simulink subsystem "PvtSubSys_PLAN_DPC"  (R2020b)
settings: Solver=VariableStepAuto  StartTime=0.0  StopTime=10.0  RelTol=1e-3
undefined symbols (not defined in the file or in its folder): P_Global_DxvFrontBumper_m, P_Global_DxvRearBumper_m, P_PLAN_DPC_BrkPointDxFactorF1, P_PLAN_DPC_BrkPointDxFactorF2, P_PLAN_DPC_BrkPointDxFactorF3, P_PLAN_DPC_BrkPointDxFactorF4, P_PLAN_DPC_BrkPointDxFactorR1, P_PLAN_DPC_BrkPointDxFactorR2, P_PLAN_DPC_BrkPointDxFactorR3, P_PLAN_DPC_BrkPointDxFactorR4, P_PLAN_DPC_danqianleida_kaiguan, P_PLAN_DPC_danqianleida_maxDx, P_PLAN_DPC_danqianleida_minDx, P_PLAN_DPC_FrontObj_DX_00, P_PLAN_DPC_FrontObj_DX_03, P_PLAN_DPC_FrontObj_DX_08, P_PLAN_DPC_FrontObj_DX_1, P_PLAN_DPC_HearObj_DX_00, P_PLAN_DPC_HearObj_DX_03, P_PLAN_DPC_HearObj_DX_08, P_PLAN_DPC_HearObj_DX_11, P_PLAN_DPC_HWALineRearA2Factor, P_PLAN_DPC_HWALineRearA3Factor, P_PLAN_DPC_ObjAxLPalpha, P_PLAN_DPC_ObjDxLPalpha, P_PLAN_DPC_ObjDyLPalpha, P_PLAN_DPC_ObjVxLPalpha, P_PLAN_DPC_xiangduisudu_kmh
libraries: simulink x22
(part 1 of 3)
settings Model: Creator=GW00166368  LastModifiedBy=GW00180587

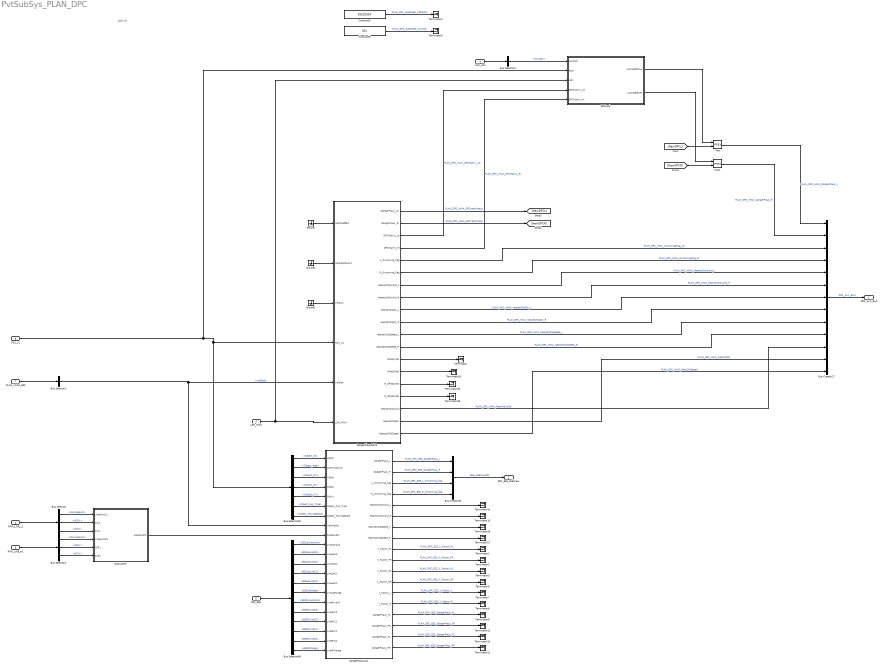
== system PvtSubSys_PLAN_DPC ==
  note: 变更记录
  VSM_HMI : Inport  Description=用了bus里面的HWASts，判断是否换道，用于锁止模块释放信号  OutDataTypeStr=Bus: VSM_HMI_BUS
  RFM_LINE_L1 : Inport  Description=本车道左车道线的属性用于计算车道宽度  Port=2  OutDataTypeStr=Bus: RFM_LINE_BUS
  RFM_LINE_R1 : Inport  Description=本车道右车道线的属性用于计算车道宽度  Port=3  OutDataTypeStr=Bus: RFM_LINE_BUS
  LSM_HWA : Inport  Description=|  Port=4  OutDataTypeStr=Bus: LSM_HWA_BUS
      | HWALeLineValid	boolean	1			HWA左目标线有效性
      | HWALeLineC3	single	1			HWA左目标线C3
      | HWALeLineC2	single	1			HWA左目标线C2
      | HWALeLineC1	single	1			HWA左目标线C1
      | HWALeLineC0	single	1			HWA左目标线C0
      | HWALeRange	single	1			HWA左目标线有效长度
      | HWALineValid	boolean	1			HWA目标线有效性
      | HWALineC3	single	1			HWA目标线C3
      | HWALineC2	single	1			HWA目标线C2
      | HWALineC1	single	1			HWA目标线C1
      | HWALineC0	single	1			HWA目标线C0
      | HWARange	single	1	m		HWA目标线有效长度
      | HWARiLineValid	boolean	1			HWA右目标线有效性
      | HWARiLineC3	single	1			HWA右目标线C3
      | HWARiLineC2	single	1			HWA右目标线C2
      | HWARiLineC1	single	1			HWA右目标线C1
      | HWARiLineC0	single	1			HWA右目标线C0
      | HWARiRange	single	1			HWA右目标线有效长度
  LSM_ESS : Inport  Description=|  Port=5  OutDataTypeStr=Bus: LSM_ESS_BUS
      | ESSLeLineValid	boolean	1			ESS左车道有效性
      | ESSLeLineC3	single	1			ESS左车道C3
      | ESSLeLineC2	single	1			ESS左车道C2
      | ESSLeLineC1	single	1			ESS左车道C1
      | ESSLeLineC0	single	1			ESS左车道C0
      | ESSLeRange	single	1			ESS左车道有效长度
      | ESSRiLineValid	boolean	1			ESS右车道有效性
      | ESSRiLineC3	single	1			ESS右车道C3
      | ESSRiLineC2	single	1			ESS右车道C2
      | ESSRiLineC1	single	1			ESS右车道C1
      | ESSRiLineC0	single	1			ESS右车道C0
      | ESSRiRange	single	1			ESS右车道有效长度
  TOS_LC : Inport  Description=|  Port=6  OutDataTypeStr=Bus: TOS_LC_BUS
      | Object_ID	single	(11,1)			障碍物ID。用于判断障碍物是否有效计算。
      | Object_DX	single	(11,1)			障碍物纵向距离。用于危险度计算。
      | Object_DY	single	(11,1)			障碍物横向距离。用于危险度计算。
      | Object_VX	single	(11,1)			障碍物纵向速度。用于危险度计算
  PLAN_VCAN_ESP : Inport  Description=自车车速  Port=7  OutDataTypeStr=Bus: VCAN_ESP_MSG_BUS
  Bus Creator17 : BusCreator  Inputs=13
  Bus Creator30 : BusCreator  Inputs=4
  Bus Selector : BusSelector  OutputSignals=bIsLineExist,dC0V,dC1V
  Bus Selector1 : BusSelector  OutputSignals=bIsLineExist,dC0V,dC1V
  Bus Selector2 : BusSelector  OutputSignals=VehSpd
  Bus Selector3 : BusSelector  OutputSignals=HWASts
  Bus Selector68 : BusSelector  OutputSignals=ESSLeLineValid,ESSLeLineC3,ESSLeLineC2,ESSLeLineC1,ESSLeLineC0,ESSLeRange,ESSRiLineValid,ESSRiLineC3,ESSRiLineC2,ESSRiLineC1,ESSRiLineC0,ESSRiRange
  Bus Selector82 : BusSelector  OutputSignals=Object_ID,Object_Age,Object_DX,Object_DY,Object_VX,Object_Fus_Type,Object_MovingState
  Constant5 : Constant  Value=39220304  OutDataTypeStr=uint32
  Constant6 : Constant  Value=301  OutDataTypeStr=uint32
  DPCLock : Subsystem
  DangerPlausCalc : Subsystem
      settings: RTWFcnNameOpts=Use subsystem name  RTWFileNameOpts=Use function name
  DangerPlausCalc3 : Subsystem
      settings: RTWFcnNameOpts=Use subsystem name  RTWFileNameOpts=Use function name
  Ground : Ground
  Ground1 : Ground
  Ground2 : Ground
  Max : MinMax  Function=max  Inputs=2  OutDataTypeStr=single
  Max1 : MinMax  Function=max  Inputs=2  OutDataTypeStr=single
  Subsystem : Subsystem
  Terminator{,1..12,14..15,26..27,31..32,39} (20 alike) : Terminator
  DPC_ALC_BUS : Outport  Description=|  OutDataTypeStr=Bus: PLAN_DPC_ALC_BUS
      | DangerPlaus_Ri	single	1			右侧危险度
      | R_Oncoming_flag	boolean	1			右侧对向障碍物标志位
      | NearestObjValid_R	boolean	1			右侧最近障碍物有效性
      | NearestObjDx_R	single	1	m		右侧最近障碍物纵向距离
      | NearestObjSpeed_R	single	1	m/s		右侧最近障碍物速度
      | DangerPlaus_Le	single	1			左侧危险度
      | L_Oncoming_flag	boolean	1			左侧对向障碍物标志位
      | NearestObjValid_L	boolean	1			左侧最近障碍物有效性
      | NearestObjDx_L	single	1	m		左侧最近障碍物纵向距离
      | NearestObjSpeed_L	single	1	m/s		左侧最近障碍物速度
      | DangerPlaus_Cr	single	1			本车道危险度
  DPC_ESS_SideView : Outport  Description=|  Port=2  OutDataTypeStr=Bus: PLAN_DPC_ESS_BUS
      | DangerPlaus_L	single	1			左侧车道危险度
      | DangerPlaus_R	single	1			右侧车道危险度
      | L_Oncoming_flag	boolean	1			左侧对向障碍物标志位
      | R_Oncoming_flag	boolean	1			右侧对向障碍物标志位
  wires:
  Constant5/1 -> Terminator4/1  "PLAN_DPC_SubModel_VERSION"
  Constant6/1 -> Terminator5/1  "PLAN_DPC_SubModel_Number"
  Max/1 -> Bus Creator17/1  "PLAN_DPC_HWA_DangerPlaus_L"
  Ground2/1 -> DangerPlausCalc3/3(VehAcc)
  DPCLock/2(LockedDPCRi) -> Max1/1
  DangerPlausCalc3/3(DPCMatrix_Le) -> DPCLock/4(DPCMatrix_Le)  "PLAN_DPC_HWA_DPCMatrix_Le"
  DangerPlausCalc3/11(NearestObjSpeed_L) -> Bus Creator17/9  "PLAN_DPC_HWA_NearestObjSpeed_L"
  DangerPlausCalc/11(X_Factor_RL) -> Terminator3/1  "PLAN_DPC_ESS_X_Factor_RL"
  DangerPlausCalc/12(X_Factor_RR) -> Terminator6/1  "PLAN_DPC_ESS_X_Factor_RR"
  Ground/1 -> DangerPlausCalc3/1(velPlanEffect)
  DangerPlausCalc/1(DangerPlaus_L) -> Bus Creator30/1  "PLAN_DPC_ESS_DangerPlaus_L"
  TOS_LC/1 -> DangerPlausCalc3/4(TOS_LC), Bus Selector82/1, DPCLock/2(TOS)
  DangerPlausCalc3/18(NearestObjDx) -> Bus Creator17/12  "PLAN_DPC_HWA_RearObjDx"
  [NewDPCR] -> Max1/2
  DangerPlausCalc/13(Y_Factor_L) -> Terminator7/1  "PLAN_DPC_ESS_Y_Factor_L"
  Bus Selector1/2 -> Subsystem/5(C0R1)  "<dC0V>"
  Bus Selector82/5 -> DangerPlausCalc/5(ObjVx)  "<Object_VX>"
  LSM_HWA/1 -> DangerPlausCalc3/6(LSM_HWA), DPCLock/3(LSM)
  DangerPlausCalc3/8(NearestObjValid_R) -> Bus Creator17/6  "PLAN_DPC_HWA_NearestObjValid_R"
  Bus Selector82/6 -> DangerPlausCalc/6(Object_Fus_Type)  "<Object_Fus_Type>"
  Bus Selector/3 -> Subsystem/3(C1L1)  "<dC1V>"
  DPCLock/1(LockedDPCLe) -> Max/1
  DangerPlausCalc3/10(NearestObjDx_R) -> Bus Creator17/8  "PLAN_DPC_HWA_NearestObjDx_R"
  DangerPlausCalc3/5(L_Oncoming_flag) -> Bus Creator17/3  "PLAN_DPC_HWA_OncomingFlag_Le"
  DangerPlausCalc3/15(R_dPreDxRel) -> Terminator32/1
  VSM_HMI/1 -> Bus Selector3/1
  DangerPlausCalc3/9(NearestObjDx_L) -> Bus Creator17/7  "PLAN_DPC_HWA_NearestObjDx_L"
  DangerPlausCalc3/17(NearestObjValid) -> Bus Creator17/11  "PLAN_DPC_HWA_RearObjValid"
  DangerPlausCalc/4(R_Oncoming_flag) -> Bus Creator30/4  "PLAN_DPC_ESS_R_Oncoming_flag"
  Bus Selector68/7 -> DangerPlausCalc/16(LineRiValid)  "<ESSRiLineValid>"
  DangerPlausCalc/3(L_Oncoming_flag) -> Bus Creator30/3  "PLAN_DPC_ESS_L_Oncoming_flag"
  Ground1/1 -> DangerPlausCalc3/2(velSubjPlanArb)
  Bus Selector82/3 -> DangerPlausCalc/3(ObjDx)  "<Object_DX>"
  PLAN_VCAN_ESP/1 -> Bus Selector2/1
  DangerPlausCalc3/14(dPreDxRel) -> Terminator31/1
  Bus Selector68/5 -> DangerPlausCalc/14(LineLeC0)  "<ESSLeLineC0>"
  Bus Selector1/3 -> Subsystem/6(C1R1)  "<dC1V>"
  DangerPlausCalc3/4(DPCMatrix_Ri) -> DPCLock/5(DPCMatrix_Ri)  "PLAN_DPC_HWA_DPCMatrix_Ri"
  DangerPlausCalc/15(DangerPlaus_FL) -> Terminator9/1  "PLAN_DPC_ESS_DangerPlaus_FL"
  DangerPlausCalc/10(X_Factor_FR) -> Terminator2/1  "PLAN_DPC_ESS_X_Factor_FR"
  Bus Selector82/7 -> DangerPlausCalc/7(Object_MovingState)  "<Object_MovingState>"
  Bus Selector68/12 -> DangerPlausCalc/21(LineRiRange)  "<ESSRiRange>"
  [NewDPCL] -> Max/2
  DangerPlausCalc/9(X_Factor_FL) -> Terminator1/1  "PLAN_DPC_ESS_X_Factor_FL"
  Bus Selector68/11 -> DangerPlausCalc/20(LineRiC0)  "<ESSRiLineC0>"
  DangerPlausCalc3/19(NearestObjSpeed) -> Bus Creator17/13  "PLAN_DPC_HWA_RearObjSpeed"
  Bus Selector68/10 -> DangerPlausCalc/19(LineRiC1)  "<ESSRiLineC1>"
  Bus Selector68/2 -> DangerPlausCalc/11(LineLeC3)  "<ESSLeLineC3>"
  Max1/1 -> Bus Creator17/2  "PLAN_DPC_HWA_DangerPlaus_R"
  DangerPlausCalc3/12(NearestObjSpeed_R) -> Bus Creator17/10  "PLAN_DPC_HWA_NearestObjSpeed_R"
  RFM_LINE_L1/1 -> Bus Selector/1
  Bus Selector68/8 -> DangerPlausCalc/17(LineRiC3)  "<ESSRiLineC3>"
  DangerPlausCalc3/2(DangerPlaus_Ri) -> [NewDPCR]  "PLAN_DPC_HWA_DPCrealtimeRi"
  Bus Selector1/1 -> Subsystem/4(LineExistR1)  "<bIsLineExist>"
  Bus Creator30/1 -> DPC_ESS_SideView/1  "ESS_SideViewSts"
  DangerPlausCalc/17(DangerPlaus_RL) -> Terminator10/1  "PLAN_DPC_ESS_DangerPlaus_RL"
  Bus Selector68/3 -> DangerPlausCalc/12(LineLeC2)  "<ESSLeLineC2>"
  Bus Selector68/4 -> DangerPlausCalc/13(LineLeC1)  "<ESSLeLineC1>"
  Bus Selector3/1 -> DPCLock/1(HWASts)  "<HWASts>"
  DangerPlausCalc3/16(R_dPreDyRel) -> Terminator39/1
  RFM_LINE_R1/1 -> Bus Selector1/1
  DangerPlausCalc/6(NearestObjValid_R) -> Terminator15/1
  Bus Selector68/6 -> DangerPlausCalc/15(LineLeRange)  "<ESSLeRange>"
  Bus Selector/2 -> Subsystem/2(C0L1)  "<dC0V>"
  DangerPlausCalc3/7(NearestObjValid_L) -> Bus Creator17/5  "PLAN_DPC_HWA_NearestObjValid_L"
  Bus Selector/1 -> Subsystem/1(LineExistL1)  "<bIsLineExist>"
  Bus Selector82/4 -> DangerPlausCalc/4(ObjDy)  "<Object_DY>"
  DangerPlausCalc/8(NearestObjSpeed_R) -> Terminator27/1
  Bus Creator17/1 -> DPC_ALC_BUS/1  "DPC_ALC_BUS"
  DangerPlausCalc/14(Y_Factor_R) -> Terminator8/1  "PLAN_DPC_ESS_Y_Factor_R"
  DangerPlausCalc3/1(DangerPlaus_Le) -> [NewDPCL]  "PLAN_DPC_HWA_DPCrealtimeLe"
  DangerPlausCalc/18(DangerPlaus_RR) -> Terminator11/1  "PLAN_DPC_ESS_DangerPlaus_RR"
  Bus Selector68/9 -> DangerPlausCalc/18(LineRiC2)  "<ESSRiLineC2>"
  DangerPlausCalc3/6(R_Oncoming_flag) -> Bus Creator17/4  "PLAN_DPC_HWA_OncomingFlag_Ri"
  DangerPlausCalc/16(DangerPlaus_FR) -> Terminator12/1  "PLAN_DPC_ESS_DangerPlaus_FR"
  DangerPlausCalc/7(NearestObjSpeed_L) -> Terminator26/1
  Subsystem/1(RoadWidth) -> DangerPlausCalc/9(RoadWidth)
  DangerPlausCalc/2(DangerPlaus_R) -> Bus Creator30/2  "PLAN_DPC_ESS_DangerPlaus_R"
  DangerPlausCalc3/13(dPreDyRel) -> Terminator/1
  DangerPlausCalc/5(NearestObjValid_L) -> Terminator14/1
  Bus Selector82/1 -> DangerPlausCalc/1(ObjID)  "<Object_ID>"
  Bus Selector68/1 -> DangerPlausCalc/10(LineLeValid)  "<ESSLeLineValid>"
  Bus Selector82/2 -> DangerPlausCalc/2(ObjTimeAlive)  "<Object_Age>"
  Bus Selector2/1 -> DangerPlausCalc3/5(VehSpd), DangerPlausCalc/8(VehicleSts)  "<VehSpd>"
  LSM_ESS/1 -> Bus Selector68/1

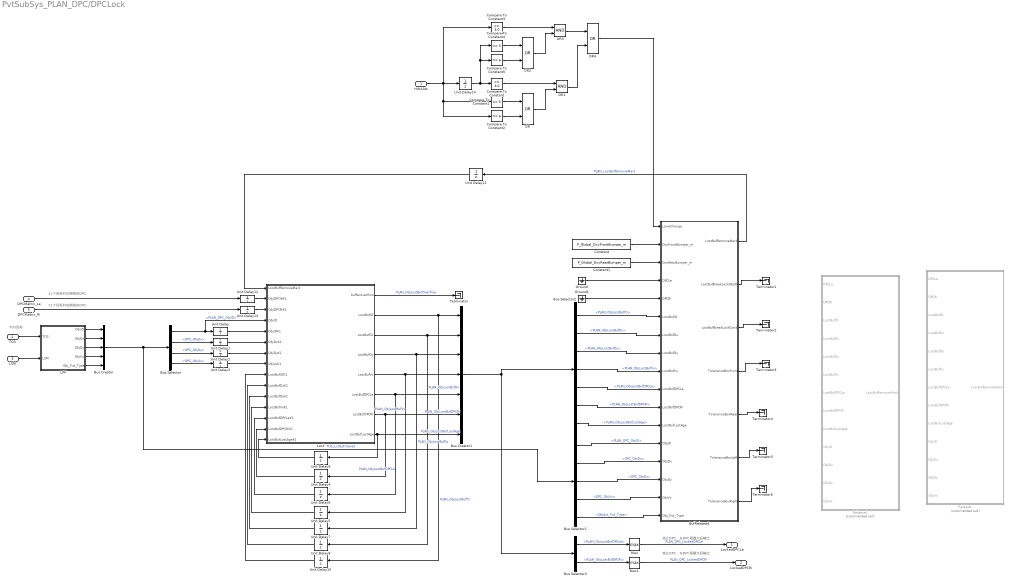
== system PvtSubSys_PLAN_DPC/DPCLock ==
  note: 锁止DPC，与DPC取最大后输出
  note: TOS目标
  note: 11个目标对右侧线的DPC
  note: 11个目标对左侧线的DPC
  note: 锁止DPC，与DPC取最大后输出
  HWASts : Inport
  TOS : Inport  Port=2
  LSM : Inport  Port=3
  DPCMatrix_Le : Inport  Port=4
  DPCMatrix_Ri : Inport  Port=5
  BufRelease1 : MATLAB Function  TreatAsAtomicUnit=on
  Bus Creator1 : BusCreator  Inputs=7
  Bus Selector : BusSelector  OutputSignals=PLAN_DPC_ObjID,DPC_ObjDx,DPC_ObjDy,DPC_ObjVx
  Bus Selector1 : BusSelector  OutputSignals=PLAN_DPC_ObjID,DPC_ObjDx,DPC_ObjDy,DPC_ObjVx,Object_Fus_Type
  Bus Selector2 : BusSelector  OutputSignals=PLAN_ObjLostBufID,PLAN_ObjLostBufDx,PLAN_ObjLostBufDy,PLAN_ObjLostBufVx,PLAN_ObjLostBufDPCLe,PLAN_ObjLostBufDPCRi,PLAN_ObjLostBufLostAge
  Bus Selector3 : BusSelector  OutputSignals=PLAN_ObjLostBufDPCLe,PLAN_ObjLostBufDPCRi
  Bus Creator : BusCreator  Inputs=5
  Compare To Constant : simulink/Logic and Bit Operations/Compare To Constant  relop===  const=3.0  OutDataTypeStr=boolean
  Compare To Constant1 : simulink/Logic and Bit Operations/Compare To Constant  relop===  const=5  OutDataTypeStr=boolean
  Compare To Constant2 : simulink/Logic and Bit Operations/Compare To Constant  relop===  const=6  OutDataTypeStr=boolean
  Compare To Constant3 : simulink/Logic and Bit Operations/Compare To Constant  relop===  const=3.0  OutDataTypeStr=boolean
  Compare To Constant4 : simulink/Logic and Bit Operations/Compare To Constant  relop===  const=5  OutDataTypeStr=boolean
  Compare To Constant5 : simulink/Logic and Bit Operations/Compare To Constant  relop===  const=6  OutDataTypeStr=boolean
  Constant : Constant  Value=P_Global_DxvFrontBumper_m
  Constant1 : Constant  Value=P_Global_DxvRearBumper_m
  Ground : Ground
  Ground1 : Ground
  LPF : Subsystem
  Lock : MATLAB Function  TreatAsAtomicUnit=on
  Max : MinMax  Function=max
  Max1 : MinMax  Function=max
  OR : Logic  Operator=OR  AllPortsSameDT=off  OutDataTypeStr=boolean
  OR1 : Logic  AllPortsSameDT=off  OutDataTypeStr=boolean
  OR2 : Logic  Operator=OR  AllPortsSameDT=off  OutDataTypeStr=boolean
  OR3 : Logic  AllPortsSameDT=off  OutDataTypeStr=boolean
  OR4 : Logic  Operator=OR  AllPortsSameDT=off  OutDataTypeStr=boolean
  Release : MATLAB Function  Commented=on  TreatAsAtomicUnit=on
  Release1 : MATLAB Function  Commented=on  TreatAsAtomicUnit=on
  Terminator{,1..6} (7 alike) : Terminator
  Unit Delay{,1..3,12..14} (7 alike) : UnitDelay  SampleTime=-1  HasFrameUpgradeWarning=on
  Unit Delay{4..10} (7 alike) : UnitDelay  InitialCondition=single(zeros(11,1))  SampleTime=-1  HasFrameUpgradeWarning=on
  Unit Delay11 : UnitDelay  InitialCondition=uint8(zeros(11,1))  SampleTime=-1  HasFrameUpgradeWarning=on
  LockedDPCLe : Outport
  LockedDPCRi : Outport  Port=2
  wires:
  Bus Selector1/5 -> BufRelease1/17(Obj_Fus_Type)  "<Object_Fus_Type>"
  LPF/5(Obj_Fus_Type) -> Bus Creator/5
  Unit Delay13/1 -> Lock/3(ObjDPCRiK1)
  Unit Delay12/1 -> Lock/2(ObjDPCleK1)
  DPCMatrix_Ri/1 -> Unit Delay13/1
  DPCMatrix_Le/1 -> Unit Delay12/1
  Max1/1 -> LockedDPCRi/1  "PLAN_DPC_LockedDPCRi"
  Max/1 -> LockedDPCLe/1  "PLAN_DPC_LockedDPCLe"
  Bus Selector3/2 -> Max1/1  "<PLAN_ObjLostBufDPCRi>"
  Bus Selector3/1 -> Max/1  "<PLAN_ObjLostBufDPCLe>"
  Bus Selector2/7 -> BufRelease1/12(LostBufLostAge)  "<PLAN_ObjLostBufLostAge>"
  Bus Selector2/6 -> BufRelease1/11(LostBufDPCRi)  "<PLAN_ObjLostBufDPCRi>"
  Bus Selector2/1 -> BufRelease1/6(LostBufID)  "<PLAN_ObjLostBufID>"
  Bus Selector2/5 -> BufRelease1/10(LostBufDPCLe)  "<PLAN_ObjLostBufDPCLe>"
  Bus Selector2/2 -> BufRelease1/7(LostBufDx)  "<PLAN_ObjLostBufDx>"
  Bus Selector2/4 -> BufRelease1/9(LostBufVx)  "<PLAN_ObjLostBufVx>"
  Bus Selector2/3 -> BufRelease1/8(LostBufDy)  "<PLAN_ObjLostBufDy>"
  Ground1/1 -> BufRelease1/5(DPCRi)
  Ground/1 -> BufRelease1/4(DPCLe)
  Bus Creator1/1 -> Bus Selector2/1, Bus Selector3/1
  Lock/1(bufferoverflow) -> Terminator/1  "PLAN_ObjLostBufOverflow"
  Unit Delay10/1 -> Lock/9(LostBufIDK1)
  Unit Delay8/1 -> Lock/10(LostBufDxK1)
  Unit Delay7/1 -> Lock/11(LostBufDyK1)
  Unit Delay6/1 -> Lock/13(LostBufDPCLeK1)
  Unit Delay5/1 -> Lock/12(LostBufVxK1)
  Unit Delay4/1 -> Lock/14(LostBufDPCRiK1)
  Lock/7(LostBufDPCRi) -> Bus Creator1/6, Unit Delay4/1  "PLAN_ObjLostBufDPCRi"
  Lock/6(LostBufDPCLe) -> Bus Creator1/5, Unit Delay6/1  "PLAN_ObjLostBufDPCLe"
  Bus Selector1/4 -> BufRelease1/16(ObjVx)  "<DPC_ObjVx>"
  Bus Selector1/3 -> BufRelease1/15(ObjDy)  "<DPC_ObjDy>"
  Bus Selector1/2 -> BufRelease1/14(ObjDx)  "<DPC_ObjDx>"
  Bus Selector1/1 -> BufRelease1/13(ObjID)  "<PLAN_DPC_ObjID>"
  Unit Delay11/1 -> Lock/1(LostBufRemoveMark)
  BufRelease1/1(LostBufRemoveMark) -> Unit Delay11/1  "PLAN_LostBufRemoveMark"
  Bus Selector/1 -> Unit Delay/1, Lock/4(ObjID)  "<PLAN_DPC_ObjID>"
  Bus Selector/4 -> Unit Delay3/1  "<DPC_ObjVx>"
  Bus Selector/2 -> Unit Delay1/1  "<DPC_ObjDx>"
  Bus Selector/3 -> Unit Delay2/1  "<DPC_ObjDy>"
  Bus Creator/1 -> Bus Selector/1, Bus Selector1/1  "TOS_LcObjFiltered"
  LPF/4(ObjVx) -> Bus Creator/4
  LPF/3(ObjDy) -> Bus Creator/3
  LPF/2(ObjDx) -> Bus Creator/2
  LPF/1(ObjID) -> Bus Creator/1
  TOS/1 -> LPF/1(TOS)
  Unit Delay9/1 -> Lock/15(LostBufLostAgeK1)
  Lock/8(LostBufLostAge) -> Bus Creator1/7, Unit Delay9/1  "PLAN_ObjLostBufLostAge"
  Lock/5(LostBufVx) -> Bus Creator1/4, Unit Delay5/1  "PLAN_ObjLostBufVx"
  Lock/4(LostBufDy) -> Bus Creator1/3, Unit Delay7/1  "PLAN_ObjLostBufDy"
  Lock/3(LostBufDx) -> Bus Creator1/2, Unit Delay8/1  "PLAN_ObjLostBufDx"
  Lock/2(LostBufID) -> Bus Creator1/1, Unit Delay10/1  "PLAN_ObjLostBufID"
  Unit Delay3/1 -> Lock/8(ObjVxK1)
  Unit Delay2/1 -> Lock/7(ObjDyK1)
  Unit Delay1/1 -> Lock/6(ObjDxK1)
  Unit Delay/1 -> Lock/5(ObjIDK1)
  LSM/1 -> LPF/2(LSM)
  Constant/1 -> BufRelease1/2(DxvFrontBumper_m)
  Constant1/1 -> BufRelease1/3(DxvRearBumper_m)
  BufRelease1/2(LostBufBreakLockObjID) -> Terminator1/1
  BufRelease1/3(LostBufBreakLockCond) -> Terminator2/1
  BufRelease1/4(ToleranceBoxFront) -> Terminator3/1
  BufRelease1/5(ToleranceBoxRear) -> Terminator4/1
  BufRelease1/6(ToleranceBoxLeft) -> Terminator5/1
  BufRelease1/7(ToleranceBoxRight) -> Terminator6/1
  OR1/1 -> OR4/2
  Compare To Constant1/1 -> OR/1
  Compare To Constant2/1 -> OR/2
  Compare To Constant/1 -> OR1/1
  OR/1 -> OR1/2
  OR2/1 -> OR3/2
  Compare To Constant3/1 -> OR3/1
  Compare To Constant5/1 -> OR2/2
  Compare To Constant4/1 -> OR2/1
  HWASts/1 -> Unit Delay14/1, Compare To Constant3/1, Compare To Constant2/1, Compare To Constant1/1
  Unit Delay14/1 -> Compare To Constant4/1, Compare To Constant5/1, Compare To Constant/1
  OR3/1 -> OR4/1
  OR4/1 -> BufRelease1/1(LaneChange)

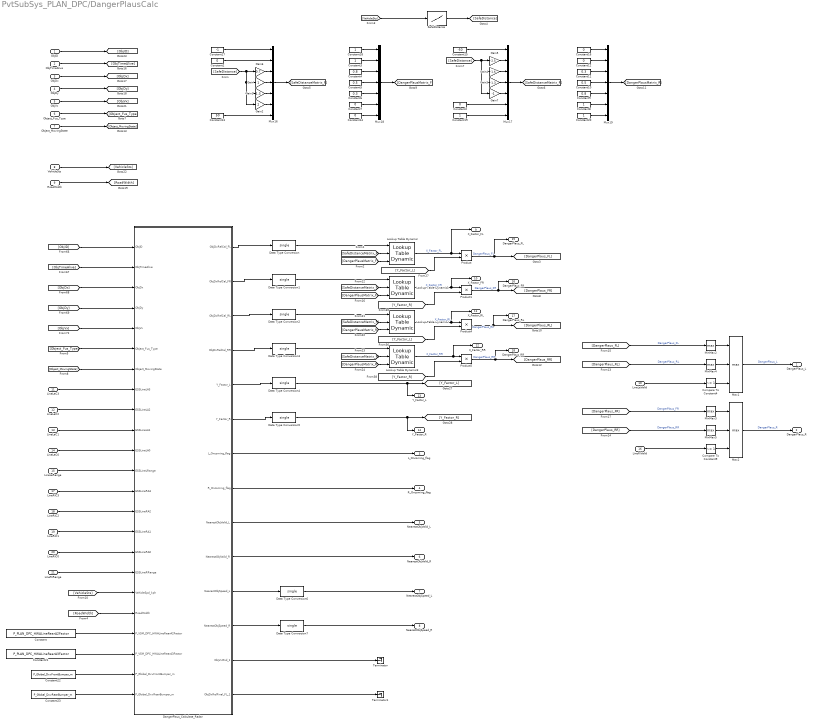
== system PvtSubSys_PLAN_DPC/DangerPlausCalc ==
  ObjID : Inport  PortDimensions=11
  ObjTimeAlive : Inport  Port=2  PortDimensions=11
  ObjDx : Inport  Port=3  PortDimensions=11
  ObjDy : Inport  Port=4  PortDimensions=11
  ObjVx : Inport  Port=5  PortDimensions=11
  Object_Fus_Type : Inport  Port=6  PortDimensions=11
  Object_MovingState : Inport  Port=7  PortDimensions=11
  VehicleSts : Inport  Port=8
  RoadWidth : Inport  Port=9
  LineLeValid : Inport  Port=10
  LineLeC3 : Inport  Port=11
  LineLeC2 : Inport  Port=12
  LineLeC1 : Inport  Port=13
  LineLeC0 : Inport  Port=14
  LineLeRange : Inport  Port=15
  LineRiValid : Inport  Port=16
  LineRiC3 : Inport  Port=17
  LineRiC2 : Inport  Port=18
  LineRiC1 : Inport  Port=19
  LineRiC0 : Inport  Port=20
  LineRiRange : Inport  Port=21
  Compare To Constant4 : simulink/Logic and Bit Operations/Compare To Constant  relop=~=  const=1  OutDataTypeStr=uint8
  Compare To Constant9 : simulink/Logic and Bit Operations/Compare To Constant  relop=~=  const=1  OutDataTypeStr=uint8
  Constant : Constant  Value=P_PLAN_DPC_HWALineRearA2Factor
  Constant{1..2,7,12,14,16} (6 alike) : Constant  Value=0  OutDataTypeStr=Inherit: Inherit via back propagation
  Constant10 : Constant  Value=0.5  OutDataTypeStr=Inherit: Inherit via back propagation
  Constant11 : Constant  Value=0.3  OutDataTypeStr=Inherit: Inherit via back propagation
  Constant13 : Constant  Value=50  OutDataTypeStr=Inherit: Inherit via back propagation
  Constant15 : Constant  Value=-50  OutDataTypeStr=Inherit: Inherit via back propagation
  Constant17 : Constant  Value=-1  OutDataTypeStr=Inherit: Inherit via back propagation
  Constant{3,8,18..20} (5 alike) : Constant  OutDataTypeStr=Inherit: Inherit via back propagation
  Constant21 : Constant  Value=P_PLAN_DPC_HWALineRearA3Factor
  Constant22 : Constant  Value=P_Global_DxvFrontBumper_m
  Constant23 : Constant  Value=P_Global_DxvRearBumper_m
  Constant4 : Constant  Value=0.8  OutDataTypeStr=Inherit: Inherit via back propagation
  Constant5 : Constant  Value=0.5  OutDataTypeStr=Inherit: Inherit via back propagation
  Constant6 : Constant  Value=0.3  OutDataTypeStr=Inherit: Inherit via back propagation
  Constant9 : Constant  Value=0.8  OutDataTypeStr=Inherit: Inherit via back propagation
  DangerPlaus_Calculate_Radar : MATLAB Function  TreatAsAtomicUnit=on
  Data Type Conversion{,1..7} (8 alike) : DataTypeConversion  OutDataTypeStr=single
  Gain : Gain
  Gain1 : Gain  Gain=1.3
  Gain2 : Gain  Gain=2
  Gain3 : Gain  Gain=-1.3
  Gain4 : Gain  Gain=-1.6
  Gain5 : Gain  Gain=-2.5
  Gain6 : Gain  Gain=0.7
  Gain7 : Gain  Gain=-1
  Lookup Table Dynamic{,1..3} (4 alike) : simulink/Lookup Tables/Lookup Table Dynamic  LookUpMeth=Interpolation-Use End Values  OutDataType=fixdt('single')  OutScaling=[]  OutputDataTypeScalingMode=Specify via dialog  OutDataTypeStr=single  DoSatur=off
  Max1 : MinMax  Function=max  Inputs=3
  Max2 : MinMax  Function=max  Inputs=3
  MinMax{2..5} (4 alike) : MinMax  Function=max
  Mux{16..19} (4 alike) : Mux  Inputs=7
  Product{,1,4..5} (4 alike) : Product
  SafeDistance : Lookup_n-D  NumberOfTableDimensions=1  BreakpointsForDimension1=[0,20,30,40,120]  Table=[4,5,8,10,10]  RndMeth=Simplest  InputSameDT=on
  Terminator : Terminator
  Terminator1 : Terminator
  DangerPlaus_L : Outport  OutDataTypeStr=single
  DangerPlaus_R : Outport  Port=2  OutDataTypeStr=single
  L_Oncoming_flag : Outport  Port=3  OutDataTypeStr=boolean
  R_Oncoming_flag : Outport  Port=4  OutDataTypeStr=boolean
  NearestObjValid_L : Outport  Port=5  OutDataTypeStr=boolean
  NearestObjValid_R : Outport  Port=6  OutDataTypeStr=boolean
  NearestObjSpeed_L : Outport  Port=7  OutDataTypeStr=single
  NearestObjSpeed_R : Outport  Port=8  OutDataTypeStr=single
  X_Factor_FL : Outport  Port=9  OutDataTypeStr=single
  X_Factor_FR : Outport  Port=10  OutDataTypeStr=single
  X_Factor_RL : Outport  Port=11  OutDataTypeStr=single
  X_Factor_RR : Outport  Port=12  OutDataTypeStr=single
  Y_Factor_L : Outport  Port=13  OutDataTypeStr=single
  Y_Factor_R : Outport  Port=14  OutDataTypeStr=single
  DangerPlaus_FL : Outport  Port=15  OutDataTypeStr=single
  DangerPlaus_FR : Outport  Port=16  OutDataTypeStr=single
  DangerPlaus_RL : Outport  Port=17  OutDataTypeStr=single
  DangerPlaus_RR : Outport  Port=18  OutDataTypeStr=single
  wires:
  Data Type Conversion7/1 -> NearestObjSpeed_R/1
  Data Type Conversion6/1 -> NearestObjSpeed_L/1
  Data Type Conversion5/1 -> [Y_Factor_R], Y_Factor_R/1
  Data Type Conversion4/1 -> Y_Factor_L/1, [Y_Factor_L]
  Data Type Conversion3/1 -> Lookup Table Dynamic3/1
  Data Type Conversion2/1 -> Lookup Table Dynamic2/1
  Data Type Conversion1/1 -> Lookup Table Dynamic1/1
  Data Type Conversion/1 -> Lookup Table Dynamic/1
  DangerPlaus_Calculate_Radar/8(R_Oncoming_flag) -> R_Oncoming_flag/1
  DangerPlaus_Calculate_Radar/7(L_Oncoming_flag) -> L_Oncoming_flag/1
  LineRiRange/1 -> DangerPlaus_Calculate_Radar/17(ESSLineRRange)
  LineLeRange/1 -> DangerPlaus_Calculate_Radar/12(ESSLineLRange)
  [Object_Fus_Type] -> DangerPlaus_Calculate_Radar/6(Object_Fus_Type)
  [Object_MovingState] -> DangerPlaus_Calculate_Radar/7(Object_MovingState)
  Object_MovingState/1 -> [Object_MovingState]
  Object_Fus_Type/1 -> [Object_Fus_Type]
  [RoadWidth] -> DangerPlaus_Calculate_Radar/19(RoadWidth)
  [VehicleSts] -> DangerPlaus_Calculate_Radar/18(VehicleSpd_kph)
  LineRiC0/1 -> DangerPlaus_Calculate_Radar/16(ESSLineRA0)
  LineRiC1/1 -> DangerPlaus_Calculate_Radar/15(ESSLineRA1)
  LineRiC2/1 -> DangerPlaus_Calculate_Radar/14(ESSLineRA2)
  LineRiC3/1 -> DangerPlaus_Calculate_Radar/13(ESSLineRA3)
  LineLeC0/1 -> DangerPlaus_Calculate_Radar/11(ESSLineLA0)
  LineLeC1/1 -> DangerPlaus_Calculate_Radar/10(ESSLineLA1)
  LineLeC2/1 -> DangerPlaus_Calculate_Radar/9(ESSLineLA2)
  LineLeC3/1 -> DangerPlaus_Calculate_Radar/8(ESSLineLA3)
  DangerPlaus_Calculate_Radar/14(ObjDxRelFinal_FL_1) -> Terminator1/1
  DangerPlaus_Calculate_Radar/13(ObjVxGnd_1) -> Terminator/1
  VehicleSts/1 -> [VehicleSts]
  DangerPlaus_Calculate_Radar/6(Y_Factor_R) -> Data Type Conversion5/1
  DangerPlaus_Calculate_Radar/5(Y_Factor_L) -> Data Type Conversion4/1
  RoadWidth/1 -> [RoadWidth]
  DangerPlaus_Calculate_Radar/12(NearestObjSpeed_R) -> Data Type Conversion7/1
  DangerPlaus_Calculate_Radar/11(NearestObjSpeed_L) -> Data Type Conversion6/1
  DangerPlaus_Calculate_Radar/10(NearestObjValid_R) -> NearestObjValid_R/1
  DangerPlaus_Calculate_Radar/9(NearestObjValid_L) -> NearestObjValid_L/1
  [VehicleSts] -> SafeDistance/1
  Constant12/1 -> Mux19/2
  [ObjID] -> DangerPlaus_Calculate_Radar/1(ObjID)
  Product/1 -> [DangerPlaus_FL], DangerPlaus_FL/1  "DangerPlaus_FL"
  Constant17/1 -> Mux16/1
  Gain6/1 -> Mux16/3
  [DangerPlausMatrix_F] -> Lookup Table Dynamic/3
  Product1/1 -> [DangerPlaus_FR], DangerPlaus_FR/1  "DangerPlaus_FR"
  [SafeDistance] -> Gain6/1, Gain/1, Gain2/1, Gain1/1
  [DangerPlaus_RR] -> MinMax5/1  "DangerPlaus_RR"
  LineLeValid/1 -> Compare To Constant4/1
  [DangerPlausMatrix_R] -> Lookup Table Dynamic2/3
  [ObjDy] -> DangerPlaus_Calculate_Radar/4(ObjDy)
  [ObjTimeAlive] -> DangerPlaus_Calculate_Radar/2(ObjTimeAlive)
  Mux17/1 -> [SafeDistanceMatrix_R]
  Gain5/1 -> Mux17/2
  MinMax3/1 -> Max2/1
  Constant11/1 -> Mux19/3
  DangerPlaus_Calculate_Radar/3(ObjDxRelCal_RL) -> Data Type Conversion2/1
  Constant15/1 -> Mux17/1
  SafeDistance/1 -> [SafeDistance]
  [Y_Factor_R] -> Product1/2
  Constant10/1 -> Mux19/4
  Lookup Table Dynamic2/1 -> Product4/1, X_Factor_RL/1  "X_Factor_RL"
  Constant18/1 -> Mux18/1
  [ObjVx] -> DangerPlaus_Calculate_Radar/5(ObjVx)
  [DangerPlausMatrix_F] -> Lookup Table Dynamic1/3
  Constant13/1 -> Mux16/7
  [DangerPlaus_FR] -> MinMax3/1  "DangerPlaus_FR"
  [SafeDistanceMatrix_R] -> Lookup Table Dynamic2/2
  Product5/1 -> [DangerPlaus_RR], DangerPlaus_RR/1  "DangerPlaus_RR"
  Constant1/1 -> Mux16/2
  [Y_Factor_R] -> Product5/2
  Gain4/1 -> Mux17/3
  DangerPlaus_Calculate_Radar/4(ObjDxRelCal_RR) -> Data Type Conversion3/1
  [DangerPlausMatrix_R] -> Lookup Table Dynamic3/3
  Gain3/1 -> Mux17/4
  Lookup Table Dynamic/1 -> Product/1, X_Factor_FL/1  "X_Factor_FL"
  Compare To Constant4/1 -> Max1/3
  Lookup Table Dynamic3/1 -> Product5/1, X_Factor_RR/1  "X_Factor_RR"
  Compare To Constant9/1 -> Max2/3
  [SafeDistanceMatrix_F] -> Lookup Table Dynamic/2
  DangerPlaus_Calculate_Radar/2(ObjDxRelCal_FR) -> Data Type Conversion1/1
  Max2/1 -> DangerPlaus_R/1  "DangerPlaus_R"
  MinMax2/1 -> Max1/1
  MinMax4/1 -> Max1/2
  Constant8/1 -> Mux19/6
  [Y_Factor_L] -> Product4/2
  [Y_Factor_L] -> Product/2
  Mux16/1 -> [SafeDistanceMatrix_F]
  LineRiValid/1 -> Compare To Constant9/1
  [SafeDistance] -> Gain5/1, Gain7/1, Gain3/1, Gain4/1
  [DangerPlaus_RL] -> MinMax4/1  "DangerPlaus_RL"
  Constant16/1 -> Mux19/1
  Constant9/1 -> Mux19/5
  Mux18/1 -> [DangerPlausMatrix_F]
  Gain/1 -> Mux16/4
  Lookup Table Dynamic1/1 -> Product1/1, X_Factor_FR/1  "X_Factor_FR"
  [ObjDx] -> DangerPlaus_Calculate_Radar/3(ObjDx)
  Constant3/1 -> Mux18/2
  Gain1/1 -> Mux16/5
  Constant5/1 -> Mux18/4
  [DangerPlaus_FL] -> MinMax2/1  "DangerPlaus_FL"
  [SafeDistanceMatrix_F] -> Lookup Table Dynamic1/2
  Product4/1 -> [DangerPlaus_RL], DangerPlaus_RL/1  "DangerPlaus_RL"
  Constant7/1 -> Mux18/6
  Constant14/1 -> Mux18/7
  Constant19/1 -> Mux17/7
  Gain7/1 -> Mux17/5
  Constant4/1 -> Mux18/3
  Mux19/1 -> [DangerPlausMatrix_R]
  [SafeDistanceMatrix_R] -> Lookup Table Dynamic3/2
  DangerPlaus_Calculate_Radar/1(ObjDxRelCal_FL) -> Data Type Conversion/1
  Max1/1 -> DangerPlaus_L/1  "DangerPlaus_L"
  Gain2/1 -> Mux16/6
  Constant6/1 -> Mux18/5
  MinMax5/1 -> Max2/2
  Constant2/1 -> Mux17/6
  Constant20/1 -> Mux19/7
  ObjVx/1 -> [ObjVx]
  ObjDy/1 -> [ObjDy]
  ObjDx/1 -> [ObjDx]
  ObjTimeAlive/1 -> [ObjTimeAlive]
  ObjID/1 -> [ObjID]
  Constant/1 -> DangerPlaus_Calculate_Radar/20(P_VSM_DPC_HWALineRearA2Factor)
  Constant21/1 -> DangerPlaus_Calculate_Radar/21(P_VSM_DPC_HWALineRearA3Factor)
  Constant22/1 -> DangerPlaus_Calculate_Radar/22(P_Global_DxvFrontBumper_m)
  Constant23/1 -> DangerPlaus_Calculate_Radar/23(P_Global_DxvRearBumper_m)

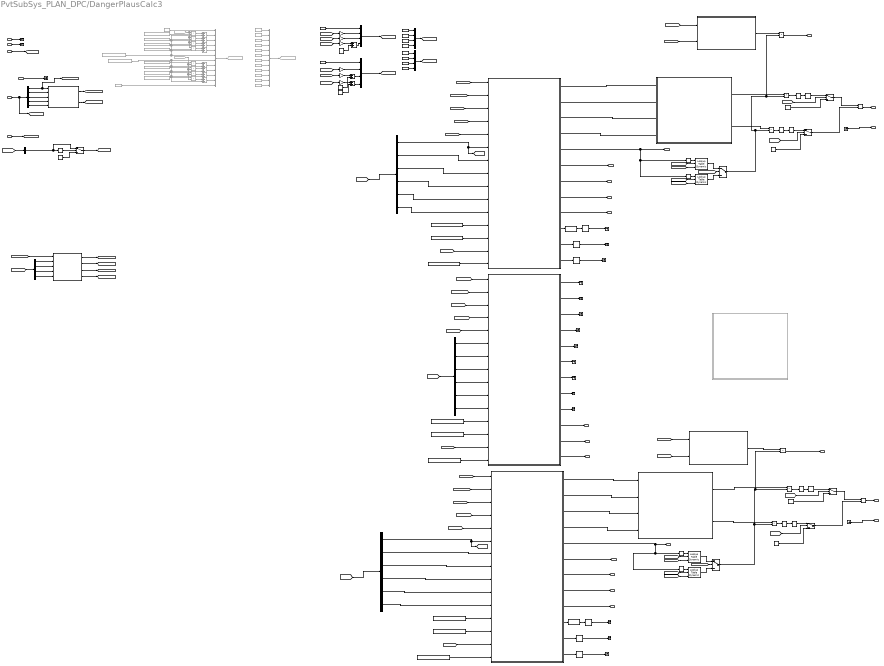
== system PvtSubSys_PLAN_DPC/DangerPlausCalc3 ==
  note: 1*11的一个数组
  note: 1*11的一个数组
  velPlanEffect : Inport
  velSubjPlanArb : Inport  Port=2
  VehAcc : Inport  Port=3
  TOS_LC : Inport  Port=4
  VehSpd : Inport  Port=5
  LSM_HWA : Inport  Port=6
  Abs{1..2,5..6} (4 alike) : Abs
  Add : Sum
  Add1 : Sum
  Add{4..11} (8 alike) : Sum  Commented=on
  Add2 : Sum
  Bus Selector : BusSelector  OutputSignals=HWALineValid,HWALineC3,HWALineC2,HWALineC1,HWALineC0,HWARange
  Bus Selector1 : BusSelector  OutputSignals=HWALeLineValid,HWALeLineC3,HWALeLineC2,HWALeLineC1,HWALeLineC0,HWALeRange
  Bus Selector2 : BusSelector  OutputSignals=Object_ID,Object_MovingState,Object_Fus_Type,Object_Age,Object_DX
  Bus Selector3 : BusSelector  OutputSignals=RoadWidth
  Bus Selector5 : BusSelector  OutputSignals=HWARiLineValid,HWARiLineC3,HWARiLineC2,HWARiLineC1,HWARiLineC0,HWARiRange
  Bus Selector7 : BusSelector  OutputSignals=Object_DX,Object_DY,Object_VX,Object_AX
  Compare To Constant2 : simulink/Logic and Bit Operations/Compare To Constant  relop=>  const=0  OutDataTypeStr=boolean
  Constant{1,17,20,37,42,46} (6 alike) : Constant  Value=0  OutDataTypeStr=Inherit: Inherit via back propagation
  Constant10 : Constant  Commented=on  Value=0.5  OutDataTypeStr=Inherit: Inherit via back propagation
  Constant11 : Constant  Commented=on  Value=0.3  OutDataTypeStr=Inherit: Inherit via back propagation
  Constant{7,12,14,16} (4 alike) : Constant  Commented=on  Value=0  OutDataTypeStr=Inherit: Inherit via back propagation
  Constant13 : Constant  Commented=on  Value=50  OutDataTypeStr=Inherit: Inherit via back propagation
  Constant15 : Constant  Commented=on  Value=-50  OutDataTypeStr=Inherit: Inherit via back propagation
  Constant18 : Constant  Value=2  OutDataTypeStr=single
  Constant{3,19,21,23,60,62} (6 alike) : Constant  OutDataTypeStr=single
  Constant2 : Constant  Commented=on  OutDataTypeStr=Inherit: Inherit via back propagation
  Constant22 : Constant  Value=P_PLAN_DPC_HWALineRearA2Factor
  Constant24 : Constant  Value=P_PLAN_DPC_HWALineRearA2Factor
  Constant25 : Constant  Value=P_PLAN_DPC_HWALineRearA3Factor
  Constant26 : Constant  Value=P_PLAN_DPC_HWALineRearA3Factor
  Constant27 : Constant  Value=11
  Constant28 : Constant  Value=11
  Constant29 : Constant  Commented=on  Value=P_PLAN_DPC_BrkPointDxFactorR4
  Constant35 : Constant  OutDataTypeStr=Inherit: Inherit via back propagation
  Constant36 : Constant  OutDataTypeStr=Inherit: Inherit via back propagation
  Constant4 : Constant  Commented=on  Value=0.8  OutDataTypeStr=Inherit: Inherit via back propagation
  Constant41 : Constant  Commented=on  Value=P_Global_DxvFrontBumper_m
  Constant43 : Constant  Commented=on  Value=P_Global_DxvRearBumper_m
  Constant44 : Constant  Value=0.6  OutDataTypeStr=Inherit: Inherit via back propagation
  Constant45 : Constant  OutDataTypeStr=Inherit: Inherit via back propagation
  Constant5 : Constant  Commented=on  Value=0.5  OutDataTypeStr=Inherit: Inherit via back propagation
  Constant6 : Constant  Commented=on  Value=0.3  OutDataTypeStr=Inherit: Inherit via back propagation
  Constant61 : Constant  Value=P_PLAN_DPC_HWALineRearA2Factor
  Constant63 : Constant  Value=P_PLAN_DPC_HWALineRearA3Factor
  Constant64 : Constant  Value=11
  Constant68 : Constant  Commented=on  Value=P_PLAN_DPC_BrkPointDxFactorR3
  Constant69 : Constant  Commented=on  Value=P_PLAN_DPC_BrkPointDxFactorR2
  Constant70 : Constant  Value=3.75  OutDataTypeStr=single
  Constant71 : Constant  Commented=on  Value=P_PLAN_DPC_BrkPointDxFactorR1
  Constant72 : Constant  Commented=on  Value=P_PLAN_DPC_BrkPointDxFactorF1
  Constant73 : Constant  Commented=on  Value=P_PLAN_DPC_BrkPointDxFactorF2
  Constant74 : Constant  Commented=on  Value=P_PLAN_DPC_BrkPointDxFactorF3
  Constant75 : Constant  Commented=on  Value=P_PLAN_DPC_BrkPointDxFactorF4
  Constant8 : Constant  Commented=on  OutDataTypeStr=Inherit: Inherit via back propagation
  Constant9 : Constant  Commented=on  Value=0.8  OutDataTypeStr=Inherit: Inherit via back propagation
  DangerFactorMatrixCalc_Left : MATLAB Function  TreatAsAtomicUnit=on
  DangerFactorMatrixCalc_Left1 : MATLAB Function  TreatAsAtomicUnit=on
  DangerFactorMatrixCalc_Left2 : MATLAB Function  TreatAsAtomicUnit=on
  Data Type Conversion1 : DataTypeConversion  OutDataTypeStr=uint8
  Data Type Conversion2 : DataTypeConversion  OutDataTypeStr=uint8
  For Iterator Subsystem1 : Subsystem  Commented=on  TreatAsAtomicUnit=on
  For Iterator Subsystem2 : Subsystem  TreatAsAtomicUnit=on
  For Iterator Subsystem4 : Subsystem  TreatAsAtomicUnit=on
  From44 : From  Commented=on  GotoTag=SafeDistance
  From45 : From  Commented=on  GotoTag=SafeDistance
  Gain10 : Gain  Gain=0.6
  Gain11 : Gain  Gain=0.5
  Gain12 : Gain  Gain=0.5
  Gain13 : Gain  Gain=0.5
  Gain8 : Gain  Gain=0.3
  Gain9 : Gain  Gain=0.6
  Goto5 : Goto  Commented=on  GotoTag=BrkPoint_Dx
  Goto9 : Goto  Commented=on  GotoTag=Factor_Dx
  Ground : Ground
  Ground1 : Ground
  Lookup Table Dynamic{1..4} (4 alike) : simulink/Lookup Tables/Lookup Table Dynamic  LookUpMeth=Interpolation-Use End Values  OutDataType=fixdt('single')  OutScaling=[]  OutputDataTypeScalingMode=Specify via dialog  OutDataTypeStr=single  DoSatur=off
  Max{1..5,7..9} (8 alike) : MinMax  Function=max
  Max10 : MinMax  Function=max  Inputs=2
  Max6 : MinMax  Function=max  Inputs=2
  Mux{1,5..7} (4 alike) : Mux
  Mux2 : Mux  Commented=on  Inputs=12
  Mux4 : Mux  Commented=on  Inputs=12
  Obj_front : Subsystem  TreatAsAtomicUnit=on
  Obj_front1 : Subsystem  TreatAsAtomicUnit=on
  Product{1..3,12..14} (6 alike) : Product
  Product{4..11} (8 alike) : Product  Commented=on
  Signal Copy{,1..5} (6 alike) : SignalConversion  OverrideOpt=off
  Subsystem : Subsystem
  Subsystem1 : Subsystem
  Switch1 : Switch  Criteria=u2 ~= 0
  Switch{2,4..5,7} (4 alike) : Switch  Criteria=u2 > Threshold
  Switch3 : Switch  Criteria=u2 ~= 0
  Switch6 : Switch  Criteria=u2 ~= 0
  Terminator{,1..17} (18 alike) : Terminator
  DangerPlaus_Le : Outport  OutDataTypeStr=single
  DangerPlaus_Ri : Outport  Port=2  OutDataTypeStr=single
  DPCMatrix_Le : Outport  Port=3  OutDataTypeStr=single
  DPCMatrix_Ri : Outport  Port=4  OutDataTypeStr=single
  L_Oncoming_flag : Outport  Port=5  OutDataTypeStr=boolean
  R_Oncoming_flag : Outport  Port=6  OutDataTypeStr=boolean
  NearestObjValid_L : Outport  Port=7  OutDataTypeStr=boolean
  NearestObjValid_R : Outport  Port=8  OutDataTypeStr=boolean
  NearestObjDx_L : Outport  Port=9  OutDataTypeStr=single
  NearestObjDx_R : Outport  Port=10  OutDataTypeStr=single
  NearestObjSpeed_L : Outport  Port=11  OutDataTypeStr=single
  NearestObjSpeed_R : Outport  Port=12  OutDataTypeStr=single
  dPreDyRel : Outport  Port=13
  dPreDxRel : Outport  Port=14
  R_dPreDxRel : Outport  Port=15
  R_dPreDyRel : Outport  Port=16
  NearestObjValid : Outport  Port=17  OutDataTypeStr=boolean
  NearestObjDx : Outport  Port=18  OutDataTypeStr=single
  NearestObjSpeed : Outport  Port=19  OutDataTypeStr=single
  wires:
  Bus Selector2/5 -> Subsystem/5(Object_DX)  "<Object_DX>"
  Bus Selector5/1 -> [RiLineValid], DangerFactorMatrixCalc_Left1/6(LineValid)  "<HWARiLineValid>"
  [LSM_HWA] -> Bus Selector5/1
  Bus Selector1/1 -> [LineValid], DangerFactorMatrixCalc_Left/6(LineValid)  "<HWALeLineValid>"
  [LSM_HWA] -> Bus Selector1/1
  Switch1/1 -> [RoadWidth]  "RoadWidth"
  Bus Selector3/1 -> Compare To Constant2/1, Switch1/1  "<RoadWidth>"
  Compare To Constant2/1 -> Switch1/2
  Constant70/1 -> Switch1/3
  Product13/1 -> Max8/1
  Product12/1 -> Max4/1
  VehSpd/1 -> [VehSpd]
  Max10/1 -> DangerPlaus_Ri/1
  Subsystem1/4(PLAN_DPC_ObjAx) -> [ObjAx]
  Bus Selector7/4 -> Subsystem1/5(Object_AX)  "<Object_AX>"
  Bus Selector7/3 -> Subsystem1/4(Object_VX)  "<Object_VX>"
  Bus Selector7/2 -> Subsystem1/3(Object_DY)  "<Object_DY>"
  Bus Selector7/1 -> Subsystem1/2(Object_DX)  "<Object_DX>"
  [TOS_LC] -> Bus Selector7/1
  [ObjID] -> Subsystem1/1(ObjValid)
  Bus Selector2/4 -> Subsystem/4(ObjTimeAlive)  "<Object_Age>"
  Bus Selector2/1 -> [ObjID], Subsystem/1(ObjID)  "<Object_ID>"
  Bus Selector2/3 -> Subsystem/3(Object_Fus_Type)  "<Object_Fus_Type>"
  Bus Selector2/2 -> Subsystem/2(Object_MovingState)  "<Object_MovingState>"
  TOS_LC/1 -> Bus Selector2/1, [TOS_LC]
  Subsystem1/3(PLAN_DPC_ObjVx) -> [ObjVx]
  Subsystem1/2(PLAN_DPC_ObjDy) -> [ObjDy]
  Subsystem1/1(PLAN_DPC_ObjDx) -> [ObjDx]
  [LSM_HWA] -> Bus Selector3/1
  Mux1/1 -> [Factor_Dy_cr]
  Constant45/1 -> Mux1/1
  Constant44/1 -> Mux1/2
  Constant42/1 -> Mux1/3
  Constant46/1 -> Mux1/4
  Subsystem/2(ObjValid) -> [ObjValid]
  LSM_HWA/1 -> [LSM_HWA]
  Add4/1 -> Mux4/8
  Constant41/1 -> Mux4/7, Add4/2, Add6/2, Add7/2, Add5/2
  Add5/1 -> Mux4/9
  Add6/1 -> Mux4/10
  Add7/1 -> Mux4/11
  Add11/1 -> Mux4/5
  Add10/1 -> Mux4/4
  Add9/1 -> Mux4/3
  Constant15/1 -> Mux4/1
  Gain12/1 -> Mux6/2
  Gain9/1 -> Mux5/3
  Gain8/1 -> Mux5/2
  Subsystem/1(ObjStationaryFlag) -> [ObjStationaryFlag]
  Mux5/1 -> [BrkPoint_Dy_S]
  Constant37/1 -> Mux7/4
  Constant20/1 -> Mux7/3
  Constant35/1 -> Mux7/2
  Constant36/1 -> Mux7/1
  Constant43/1 -> Mux4/6, Add11/2, Add10/2, Add9/2, Add8/2
  Constant14/1 -> Mux2/12
  Constant7/1 -> Mux2/11
  Constant6/1 -> Mux2/10
  Constant5/1 -> Mux2/9
  Constant4/1 -> Mux2/8
  Constant2/1 -> Mux2/7
  Constant8/1 -> Mux2/6
  Constant9/1 -> Mux2/5
  Constant10/1 -> Mux2/4
  Constant11/1 -> Mux2/3
  Constant12/1 -> Mux2/2
  Constant16/1 -> Mux2/1
  Mux7/1 -> [Factor_Dy]
  Mux6/1 -> [BrkPoint_Dy_NS]
  Constant19/1 -> Add2/2
  Add2/1 -> Mux6/3
  Constant17/1 -> Mux6/1
  [RoadWidth] -> Gain12/1
  Gain13/1 -> Add2/1
  [RoadWidth] -> Gain13/1
  [RoadWidth] -> Gain11/1
  Gain11/1 -> Add1/1
  Constant18/1 -> Add1/2
  Add1/1 -> Mux6/4
  Add/1 -> Mux5/4
  Constant3/1 -> Add/2
  Gain10/1 -> Add/1
  [RoadWidth] -> Gain10/1
  [RoadWidth] -> Gain9/1
  [RoadWidth] -> Gain8/1
  Constant1/1 -> Mux5/1
  Mux2/1 -> Goto9/1  "Factor_Dx"
  Mux4/1 -> Goto5/1  "BrkPoint_Dx"
  Constant13/1 -> Mux4/12
  Add8/1 -> Mux4/2
  VehAcc/1 -> Terminator5/1
  velPlanEffect/1 -> Terminator2/1
  velSubjPlanArb/1 -> Terminator3/1
  Product4/1 -> Add8/1
  Product5/1 -> Add9/1
  Product6/1 -> Add10/1
  Product7/1 -> Add11/1
  Constant71/1 -> Product7/2
  Constant69/1 -> Product6/2
  Constant68/1 -> Product5/2
  Constant29/1 -> Product4/2
  Product8/1 -> Add4/1
  Product9/1 -> Add5/1
  Product10/1 -> Add6/1
  Product11/1 -> Add7/1
  Constant72/1 -> Product8/1
  Constant73/1 -> Product9/1
  Constant74/1 -> Product10/1
  Constant75/1 -> Product11/1
  From44/1 -> Product7/1, Product6/1, Product5/1, Product4/1
  From45/1 -> Product11/2, Product10/2, Product9/2, Product8/2
  Data Type Conversion2/1 -> Signal Copy2/1
  Signal Copy2/1 -> Terminator/1  "RearObjValid"
  Signal Copy1/1 -> Terminator1/1  "RearObjDx"
  Signal Copy/1 -> Terminator4/1  "RearObjSpdGnd"
  DangerFactorMatrixCalc_Left/12(Rear_NearestObjSpeed) -> Signal Copy/1
  DangerFactorMatrixCalc_Left/11(Rear_NearestObjDx) -> Signal Copy1/1
  DangerFactorMatrixCalc_Left/10(Rear_NearesObjValid) -> Data Type Conversion2/1
  Max5/1 -> Switch4/1  "DangerPlausR"
  Constant62/1 -> Switch4/3
  [LineValid] -> Switch4/2
  Max2/1 -> Switch2/1  "DangerPlausF"
  [LineValid] -> Switch2/2
  Constant60/1 -> Switch2/3
  DangerFactorMatrixCalc_Left/7(NearestObjValid) -> NearestObjValid_L/1
  DangerFactorMatrixCalc_Left/6(Oncoming_flag) -> L_Oncoming_flag/1
  Switch4/1 -> Max6/2  "DPC_R"
  Max3/1 -> Max5/1
  Switch2/1 -> Max6/1  "DPC_F"
  [ObjDx] -> DangerFactorMatrixCalc_Left/3(ObjDx)
  Constant63/1 -> DangerFactorMatrixCalc_Left/13(LineRearC3Factor)
  [ObjValid] -> DangerFactorMatrixCalc_Left/2(ObjValid)
  [ObjDy] -> DangerFactorMatrixCalc_Left/4(ObjDy)
  Constant61/1 -> DangerFactorMatrixCalc_Left/12(LineRearC2Factor)
  DangerFactorMatrixCalc_Left/9(NearestObjSpeed) -> NearestObjSpeed_L/1  "FrontObjSpdGnd"
  DangerFactorMatrixCalc_Left/2(obj_front_Vx) -> Obj_front/2(obj_front_Vx)
  Lookup Table Dynamic2/1 -> Switch3/3  "Factor_Dy"
  Abs5/1 -> Lookup Table Dynamic1/1
  [BrkPoint_Dy_S] -> Lookup Table Dynamic1/2
  Abs6/1 -> Lookup Table Dynamic2/1
  [BrkPoint_Dy_NS] -> Lookup Table Dynamic2/2
  [RoadWidth] -> DangerFactorMatrixCalc_Left/14(RoadWidth)
  [ObjStationaryFlag] -> Switch3/2
  DangerFactorMatrixCalc_Left/8(NearestObjDx) -> NearestObjDx_L/1  "FrontObjDx"
  Lookup Table Dynamic1/1 -> Switch3/1  "Factor_Dy"
  Constant64/1 -> DangerFactorMatrixCalc_Left/15(MaxObjNum)
  Obj_front/2(obj_Rear_sub_DPC) -> Product3/1
  [Factor_Dy] -> Lookup Table Dynamic1/3
  DangerFactorMatrixCalc_Left/3(obj_Rear_Dx) -> Obj_front/3(obj_Rear_sub_Dx)
  Obj_front/1(obj_Front_sub_DPC) -> Product2/1
  DangerFactorMatrixCalc_Left/1(obj_front_Dx) -> Obj_front/1(obj_Front_sub_Dx)
  Product2/1 -> Max1/1
  [ObjVx] -> DangerFactorMatrixCalc_Left/5(ObjVx)
  DangerFactorMatrixCalc_Left/5(PreDyRel) -> Abs6/1, Abs5/1, dPreDyRel/1  "PLAN_DPC_HWA_PreDyRel_Le"
  Product3/1 -> Max3/1
  DangerFactorMatrixCalc_Left/4(obj_Rear_Vx) -> Obj_front/4(obj_Rear_Vx)
  [Factor_Dy] -> Lookup Table Dynamic2/3
  Max1/1 -> Max2/1
  [VehSpd] -> DangerFactorMatrixCalc_Left/1(VehSpd)
  Switch3/1 -> Product3/2, Product1/2, Product2/2  "PLAN_DPC_HWA_PreDyRel_Dy_Le"
  Bus Selector1/2 -> DangerFactorMatrixCalc_Left/7(LineC3)  "<HWALeLineC3>"
  Bus Selector1/3 -> DangerFactorMatrixCalc_Left/8(LineC2)  "<HWALeLineC2>"
  Bus Selector1/4 -> DangerFactorMatrixCalc_Left/9(LineC1)  "<HWALeLineC1>"
  Bus Selector1/5 -> DangerFactorMatrixCalc_Left/10(LineC0)  "<HWALeLineC0>"
  Bus Selector1/6 -> DangerFactorMatrixCalc_Left/11(LineRange)  "<HWALeRange>"
  Max6/1 -> DangerPlaus_Le/1
  Ground/1 -> dPreDxRel/1
  Ground1/1 -> R_dPreDxRel/1
  Switch6/1 -> Product14/2, Product12/2, Product13/2  "PLAN_DPC_HWA_PreDyRel_Dy_Ri"
  [VehSpd] -> DangerFactorMatrixCalc_Left1/1(VehSpd)
  Max4/1 -> Max7/1
  [Factor_Dy] -> Lookup Table Dynamic4/3
  DangerFactorMatrixCalc_Left1/4(obj_Rear_Vx) -> Obj_front1/4(obj_Rear_Vx)
  DangerFactorMatrixCalc_Left1/5(PreDyRel) -> R_dPreDyRel/1, Abs1/1, Abs2/1  "PLAN_DPC_HWA_PreDyRel_Ri"
  [ObjVx] -> DangerFactorMatrixCalc_Left1/5(ObjVx)
  DangerFactorMatrixCalc_Left1/1(obj_front_Dx) -> Obj_front1/1(obj_Front_sub_Dx)
  Obj_front1/1(obj_Front_sub_DPC) -> Product12/1
  DangerFactorMatrixCalc_Left1/3(obj_Rear_Dx) -> Obj_front1/3(obj_Rear_sub_Dx)
  [Factor_Dy] -> Lookup Table Dynamic3/3
  Obj_front1/2(obj_Rear_sub_DPC) -> Product13/1
  Constant27/1 -> DangerFactorMatrixCalc_Left1/15(MaxObjNum)
  Lookup Table Dynamic3/1 -> Switch6/1  "Factor_Dy"
  DangerFactorMatrixCalc_Left1/8(NearestObjDx) -> NearestObjDx_R/1  "FrontObjDx"
  [ObjStationaryFlag] -> Switch6/2
  [RoadWidth] -> DangerFactorMatrixCalc_Left1/14(RoadWidth)
  [BrkPoint_Dy_NS] -> Lookup Table Dynamic4/2
  Abs2/1 -> Lookup Table Dynamic4/1
  [BrkPoint_Dy_S] -> Lookup Table Dynamic3/2
  Abs1/1 -> Lookup Table Dynamic3/1
  Lookup Table Dynamic4/1 -> Switch6/3  "Factor_Dy"
  DangerFactorMatrixCalc_Left1/2(obj_front_Vx) -> Obj_front1/2(obj_front_Vx)
  DangerFactorMatrixCalc_Left1/9(NearestObjSpeed) -> NearestObjSpeed_R/1  "FrontObjSpdGnd"
  Constant22/1 -> DangerFactorMatrixCalc_Left1/12(LineRearC2Factor)
  [ObjDy] -> DangerFactorMatrixCalc_Left1/4(ObjDy)
  [ObjValid] -> DangerFactorMatrixCalc_Left1/2(ObjValid)
  Constant26/1 -> DangerFactorMatrixCalc_Left1/13(LineRearC3Factor)
  [ObjDx] -> DangerFactorMatrixCalc_Left1/3(ObjDx)
  Switch5/1 -> Max10/1  "DPC_F"
  Max8/1 -> Max9/1
  Switch7/1 -> Max10/2  "DPC_R"
  DangerFactorMatrixCalc_Left1/6(Oncoming_flag) -> R_Oncoming_flag/1
  DangerFactorMatrixCalc_Left1/7(NearestObjValid) -> NearestObjValid_R/1
  Constant21/1 -> Switch5/3
  [RiLineValid] -> Switch5/2
  Max7/1 -> Switch5/1  "DangerPlausF"
  [RiLineValid] -> Switch7/2
  Constant23/1 -> Switch7/3
  Max9/1 -> Switch7/1  "DangerPlausR"
  DangerFactorMatrixCalc_Left1/10(Rear_NearesObjValid) -> Data Type Conversion1/1
  DangerFactorMatrixCalc_Left1/11(Rear_NearestObjDx) -> Signal Copy4/1
  DangerFactorMatrixCalc_Left1/12(Rear_NearestObjSpeed) -> Signal Copy3/1
  Signal Copy3/1 -> Terminator8/1  "RearObjSpdGnd"
  Signal Copy4/1 -> Terminator7/1  "RearObjDx"
  Signal Copy5/1 -> Terminator6/1  "RearObjValid"
  Data Type Conversion1/1 -> Signal Copy5/1
  Bus Selector5/2 -> DangerFactorMatrixCalc_Left1/7(LineC3)  "<HWARiLineC3>"
  Bus Selector5/3 -> DangerFactorMatrixCalc_Left1/8(LineC2)  "<HWARiLineC2>"
  Bus Selector5/4 -> DangerFactorMatrixCalc_Left1/9(LineC1)  "<HWARiLineC1>"
  Bus Selector5/5 -> DangerFactorMatrixCalc_Left1/10(LineC0)  "<HWARiLineC0>"
  Bus Selector5/6 -> DangerFactorMatrixCalc_Left1/11(LineRange)  "<HWARiRange>"
  [LSM_HWA] -> Bus Selector/1
  Bus Selector/1 -> DangerFactorMatrixCalc_Left2/6(LineValid)  "<HWALineValid>"
  Bus Selector/2 -> DangerFactorMatrixCalc_Left2/7(LineC3)  "<HWALineC3>"
  Bus Selector/3 -> DangerFactorMatrixCalc_Left2/8(LineC2)  "<HWALineC2>"
  Bus Selector/4 -> DangerFactorMatrixCalc_Left2/9(LineC1)  "<HWALineC1>"
  Bus Selector/5 -> DangerFactorMatrixCalc_Left2/10(LineC0)  "<HWALineC0>"
  Bus Selector/6 -> DangerFactorMatrixCalc_Left2/11(LineRange)  "<HWARange>"
  [VehSpd] -> DangerFactorMatrixCalc_Left2/1(VehSpd)
  [ObjVx] -> DangerFactorMatrixCalc_Left2/5(ObjVx)
  [ObjDy] -> DangerFactorMatrixCalc_Left2/4(ObjDy)
  [ObjValid] -> DangerFactorMatrixCalc_Left2/2(ObjValid)
  [ObjDx] -> DangerFactorMatrixCalc_Left2/3(ObjDx)
  Constant28/1 -> DangerFactorMatrixCalc_Left2/15(MaxObjNum)
  [RoadWidth] -> DangerFactorMatrixCalc_Left2/14(RoadWidth)
  Constant24/1 -> DangerFactorMatrixCalc_Left2/12(LineRearC2Factor)
  Constant25/1 -> DangerFactorMatrixCalc_Left2/13(LineRearC3Factor)
  DangerFactorMatrixCalc_Left2/10(Rear_NearesObjValid) -> NearestObjValid/1
  DangerFactorMatrixCalc_Left2/11(Rear_NearestObjDx) -> NearestObjDx/1
  DangerFactorMatrixCalc_Left2/12(Rear_NearestObjSpeed) -> NearestObjSpeed/1
  DangerFactorMatrixCalc_Left2/1(obj_front_Dx) -> Terminator9/1
  DangerFactorMatrixCalc_Left2/2(obj_front_Vx) -> Terminator10/1
  DangerFactorMatrixCalc_Left2/3(obj_Rear_Dx) -> Terminator11/1
  DangerFactorMatrixCalc_Left2/4(obj_Rear_Vx) -> Terminator12/1
  DangerFactorMatrixCalc_Left2/5(PreDyRel) -> Terminator13/1  "PreDyRel"
  DangerFactorMatrixCalc_Left2/6(Oncoming_flag) -> Terminator14/1
  DangerFactorMatrixCalc_Left2/7(NearestObjValid) -> Terminator15/1
  DangerFactorMatrixCalc_Left2/8(NearestObjDx) -> Terminator16/1  "FrontObjDx"
  DangerFactorMatrixCalc_Left2/9(NearestObjSpeed) -> Terminator17/1  "FrontObjSpdGnd"
  [ObjVx] -> For Iterator Subsystem2/1(Obj_Vx)
  [ObjDx] -> For Iterator Subsystem2/2(Obj_Dx)
  For Iterator Subsystem2/1(DPC) -> Product1/1
  Product1/1 -> DPCMatrix_Le/1
  For Iterator Subsystem4/1(DPC) -> Product14/1
  [ObjDx] -> For Iterator Subsystem4/2(Obj_Dx)
  [ObjVx] -> For Iterator Subsystem4/1(Obj_Vx)
  Product14/1 -> DPCMatrix_Ri/1

== system PvtSubSys_PLAN_DPC/Subsystem ==
  LineExistL1 : Inport
  C0L1 : Inport  Port=2
  C1L1 : Inport  Port=3
  LineExistR1 : Inport  Port=4
  C0R1 : Inport  Port=5
  C1R1 : Inport  Port=6
  RoadWidthCalc : MATLAB Function  TreatAsAtomicUnit=on
  Unit Delay1 : UnitDelay  InitialCondition=3.75  SampleTime=-1  HasFrameUpgradeWarning=on
  RoadWidth : Outport
  wires:
  C0L1/1 -> RoadWidthCalc/2(C0L1)
  C0R1/1 -> RoadWidthCalc/5(C0R1)
  RoadWidthCalc/1(RoadWidth) -> RoadWidth/1, Unit Delay1/1
  Unit Delay1/1 -> RoadWidthCalc/7(RoadWidthK1)
  LineExistR1/1 -> RoadWidthCalc/4(LaneExistR1)
  C1R1/1 -> RoadWidthCalc/6(C1R1)
  C1L1/1 -> RoadWidthCalc/3(C1L1)
  LineExistL1/1 -> RoadWidthCalc/1(LaneExistL1)

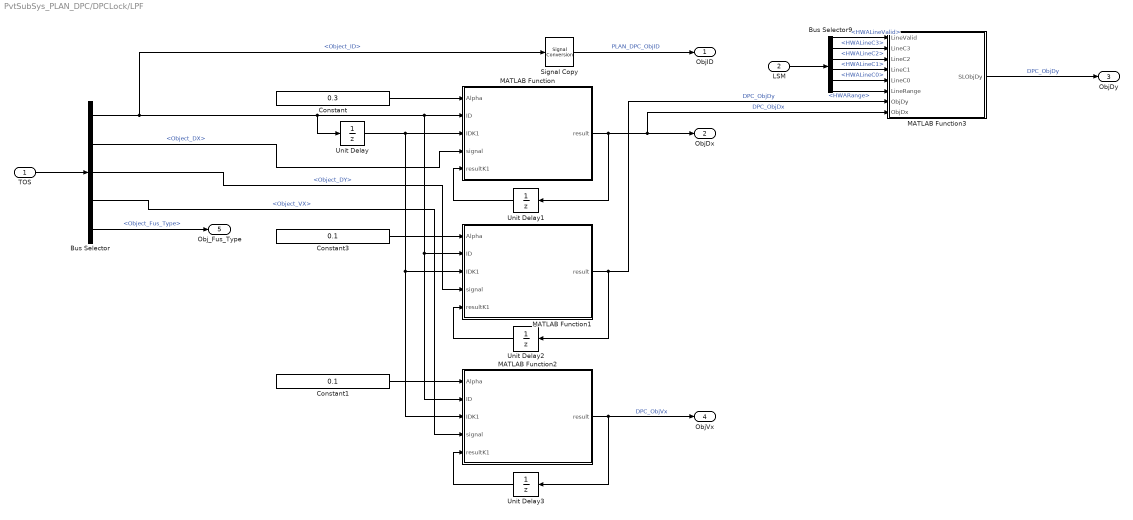
== system PvtSubSys_PLAN_DPC/DPCLock/LPF ==
  TOS : Inport
  LSM : Inport  Port=2
  Bus Selector : BusSelector  OutputSignals=Object_ID,Object_DX,Object_DY,Object_VX,Object_Fus_Type
  Bus Selector9 : BusSelector  OutputSignals=HWALineValid,HWALineC3,HWALineC2,HWALineC1,HWALineC0,HWARange
  Constant : Constant  Value=0.3
  Constant1 : Constant  Value=0.1
  Constant3 : Constant  Value=0.1
  MATLAB Function : MATLAB Function  TreatAsAtomicUnit=on
  MATLAB Function1 : MATLAB Function  TreatAsAtomicUnit=on
  MATLAB Function2 : MATLAB Function  TreatAsAtomicUnit=on
  MATLAB Function3 : MATLAB Function  TreatAsAtomicUnit=on
  Signal Copy : SignalConversion  OverrideOpt=off
  Unit Delay{,1..3} (4 alike) : UnitDelay  SampleTime=-1  HasFrameUpgradeWarning=on
  ObjID : Outport
  ObjDx : Outport  Port=2
  ObjDy : Outport  Port=3
  ObjVx : Outport  Port=4
  Obj_Fus_Type : Outport  Port=5
  wires:
  Bus Selector/5 -> Obj_Fus_Type/1  "<Object_Fus_Type>"
  MATLAB Function3/1(SLObjDy) -> ObjDy/1  "DPC_ObjDy"
  LSM/1 -> Bus Selector9/1
  Bus Selector9/6 -> MATLAB Function3/6(LineRange)  "<HWARange>"
  Bus Selector9/5 -> MATLAB Function3/5(LineC0)  "<HWALineC0>"
  Bus Selector9/4 -> MATLAB Function3/4(LineC1)  "<HWALineC1>"
  Bus Selector9/3 -> MATLAB Function3/3(LineC2)  "<HWALineC2>"
  Bus Selector9/2 -> MATLAB Function3/2(LineC3)  "<HWALineC3>"
  Bus Selector9/1 -> MATLAB Function3/1(LineValid)  "<HWALineValid>"
  Bus Selector/4 -> MATLAB Function2/4(signal)  "<Object_VX>"
  Bus Selector/2 -> MATLAB Function/4(signal)  "<Object_DX>"
  Bus Selector/1 -> Signal Copy/1, MATLAB Function1/2(ID), MATLAB Function2/2(ID), MATLAB Function/2(ID), Unit Delay/1  "<Object_ID>"
  Bus Selector/3 -> MATLAB Function1/4(signal)  "<Object_DY>"
  TOS/1 -> Bus Selector/1
  MATLAB Function2/1(result) -> Unit Delay3/1, ObjVx/1  "DPC_ObjVx"
  Constant/1 -> MATLAB Function/1(Alpha)
  Unit Delay2/1 -> MATLAB Function1/5(resultK1)
  Unit Delay/1 -> MATLAB Function1/3(IDK1), MATLAB Function2/3(IDK1), MATLAB Function/3(IDK1)
  Unit Delay1/1 -> MATLAB Function/5(resultK1)
  Unit Delay3/1 -> MATLAB Function2/5(resultK1)
  MATLAB Function1/1(result) -> MATLAB Function3/7(ObjDy), Unit Delay2/1  "DPC_ObjDy"
  Constant3/1 -> MATLAB Function1/1(Alpha)
  Constant1/1 -> MATLAB Function2/1(Alpha)
  MATLAB Function/1(result) -> ObjDx/1, MATLAB Function3/8(ObjDx), Unit Delay1/1  "DPC_ObjDx"
  Signal Copy/1 -> ObjID/1  "PLAN_DPC_ObjID"
